simulink model "Q3_M3"  (R2024b)
settings: Solver=FixedStepAuto  StartTime=0.0  StopTime=10.0  FixedStep=0.05  RelTol=1e-3
model workspace (MAT data in the model file):
  r = [0 0.1 0.2 0.3 0.4 0.5 0.6 0.7 0.8 0.9 1 1.1 1.2 1.3 1.4 1.5 1.6 1.7 1.8 1.9 2 2.1 2.2 2.3 2.4 2.5 2.6 2.7 2.8 2.9 3 3.1 3.2 3.3 3.4 3.5 3.6 3.7 3.8 3.9 4 4.1 4.2 4.3 4.4 4.5 4.6 4.7 4.8 4.9 5 5.1 5.2 5.3 5.4 5.5 5.6 5.7 5.8 5.9 6 6.1 6.2 6.3 6.4 6.5 6.6 6.7 6.8 6.9 7 7.1 7.2 7.3 7.4 7.5 7.6 7.7 7.8 7.9 8 8.1 8.2 8.3 8.4 8.5 8.6 8.7 8.8 8.9 9 9.1 9.2 9.3 9.4 9.5 9.6 9.7 9.8 9.9 10 10.1 10.2 10.3 10.4 10.5 10.6 10.7 10.8 10.9 11 11.1 11.2 11.3 11.4 11.5 11.6 11.7 11.8 11.9 12 12.1 12.2 12.3 12.4 12.5 12.6 12.7 12.8 12.9 13 13.1 13.2 13.3 13.4 13.5 13.6 13.7 13.8 13.9 14 14.1 14.2 14.3 14.4 14.5 14.6 14.7 14.8 14.9 15 15.1 15.2 15.3 15.4 15.5 15.6 15.7 15.8 15.9 16 16.1 16.2 16.3 16.4 16.5 16.6 16.7 16.8 16.9 17 17.1 17.2 17.3 17.4 17.5 17.6 17.7 17.8 17.9 18 18.1 18.2 18.3 18.4 18.5 18.6 18.7 18.8 18.9 19 19.1 19.2 19.3 19.4 19.5 19.6 19.7 19.8 19.9 20]
  theta = [0; 0.15; 0.3; 0.45; 0.6; 0.75; 0.9; 1.05; 1.2; 1.35; 1.5; 1.65; 1.8; 1.95; 2.1; 2.25; 2.4; 2.55; 2.7; 2.85; 3; 3.15; 3.3; 3.45; 3.6; 3.75; 3.9; 4.05; 4.2; 4.35; 4.5; 4.65; 4.8; 4.95; 5.1; 5.25; 5.4; 5.55; 5.7; 5.85; 6; 6.15; 6.3; 6.45; 6.6; 6.75; 6.9; 7.05; 7.2; 7.35; 7.5; 7.65; 7.8; 7.95; 8.1; 8.25; 8.4; 8.55; 8.7; 8.85; 9; 9.15; 9.3; 9.45; 9.6; 9.75; 9.9; 10.05; 10.2; 10.35; 10.5; 10.65; 10.8; 10.95; 11.1; 11.25; 11.4; 11.55; 11.7; 11.85; 12; 12.15; 12.3; 12.45; 12.6; 12.75; 12.9; 13.05; 13.2; 13.35; 13.5; 13.65; 13.8; 13.95; 14.1; 14.25; 14.4; 14.55; 14.7; 14.85; 15; 15.15; 15.3; 15.45; 15.6; 15.75; 15.9; 16.05; 16.2; 16.35; 16.5; 16.65; 16.8; 16.95; 17.1; 17.25; 17.4; 17.55; 17.7; 17.85; 18; 18.15; 18.3; 18.45; 18.6; 18.75; 18.9; 19.05; 19.2; 19.35; 19.5; 19.65; 19.8; 19.95; 20.1; 20.25; 20.4; 20.55; 20.7; 20.85; 21; 21.15; 21.3; 21.45; 21.6; 21.75; 21.9; 22.05; 22.2; 22.35; 22.5; 22.65; 22.8; 22.95; 23.1; 23.25; 23.4; 23.55; 23.7; 23.85; 24; 24.15; 24.3; 24.45; 24.6; 24.75; 24.9; 25.05; 25.2; 25.35; 25.5; 25.65; 25.8; 25.95; 26.1; 26.25; 26.4; 26.55; 26.7; 26.85; 27; 27.15; 27.3; 27.45; 27.6; 27.75; 27.9; 28.05; 28.2; 28.35; 28.5; 28.65; 28.8; 28.95; 29.1; 29.25; 29.4; 29.55; 29.7; 29.85; 30]
settings Model: Creator=chall  LastModifiedBy=chall

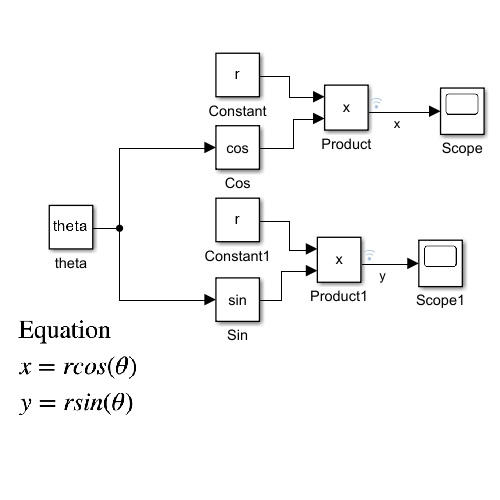
[thumbnail: Simulink's stored preview of the top-level diagram]
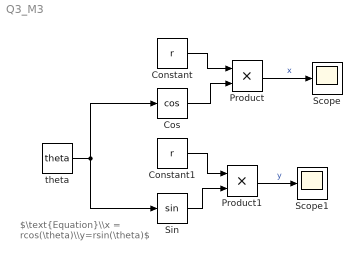
== system Q3_M3 ==
  note: $\text{Equation}\\x = rcos(\theta)\\y=rsin(\theta)$
  Constant : Constant  Value=r
  Constant1 : Constant  Value=r
  Cos : Trigonometry  Operator=cos
  Product : Product
  Product1 : Product
  Scope : Scope
  Scope1 : Scope
  Sin : Trigonometry
  theta : Constant  Value=theta
  wires:
  Constant/1 -> Product/1
  Cos/1 -> Product/2
  Constant1/1 -> Product1/1
  Sin/1 -> Product1/2
  theta/1 -> Sin/1, Cos/1
  Product/1 -> Scope/1  "x"
  Product1/1 -> Scope1/1  "y"
